simulink model "test_model"  (R2015a)
settings: Solver=ode45  StartTime=0.0  StopTime=10.0  RelTol=1e-3
settings Model: Creator=csmith  LastModifiedBy=csmith

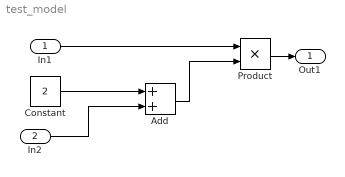
== system test_model ==
  In1 : Inport
  In2 : Inport  Port=2
  Add : Sum
  Constant : Constant  Value=2
  Product : Product
  Out1 : Outport
  wires:
  In1/1 -> Product/1
  Constant/1 -> Add/1
  In2/1 -> Add/2
  Add/1 -> Product/2
  Product/1 -> Out1/1
